simulink model "c00011M_harness"  (R2018a)
settings: Solver=FixedStepAuto  StartTime=0.0  StopTime=300  FixedStep=0.1  RelTol=1e-3
undefined symbols (not defined in the file): A1, hmax, PriorityTank, R1, R2, sigbuilder_block
(part 10 of 73)

== system c00011M_harness/M145 ==
  note: VALUES
      | ---------------------------------
      | ControlType = 1 | 2 | 3
      | FillTank = 0 | 1
      | EmptyTank = 0 | 1
      | ManualReference between 0 and 1
      | Tempreature between 0 and 100
      | EmergencyButton = 0 | 1
      | LiquidLevel between 0 and 1 (hmax)
  note: Inputs For Tank2
  note: NAMES
      | --------------------------------------------
      | CT1 = ControlType Tank 1
      | F1 = Fill Tank 1
      | E1 = Empty Tank 1
      | MR1 = Manual Reference Tank1
      | T1 = Temperature Tank 1
      | EB1 = Emergency Button Tank 1
      | LL1 = Liquid Level 1
  note: Inputs For Tank3
  note: Inputs For Tank1
  CT1 : Inport
  MR1 : Inport  Port=2
  T1 : Inport  Port=3
  EB1 : Inport  Port=4
  CT2 : Inport  Port=5
  MR2 : Inport  Port=6
  T2 : Inport  Port=7
  EB2 : Inport  Port=8
  CT3 : Inport  Port=9
  F3 : Inport  Port=10
  E3 : Inport  Port=11
  T3 : Inport  Port=12
  EB3 : Inport  Port=13
  Tank1 : Subsystem
  Tank2 : Subsystem
  Tank3 : Subsystem
  LL1 : Outport
  LL2 : Outport  Port=2
  LL3 : Outport  Port=3
  wires:
  EB1/1 -> Tank1/4(EB1)
  Tank2/1(LL2) -> LL2/1, Tank3/7(LL2), Tank1/5(LL2)
  Tank3/1(LL3) -> LL3/1, Tank2/6(LL3), Tank1/6(LL3)
  EB2/1 -> Tank2/4(EB2)
  CT2/1 -> Tank2/1(CT2)
  MR1/1 -> Tank1/2(MR1)
  T1/1 -> Tank1/3(T1)
  Tank1/1(LL1) -> LL1/1, Tank3/6(LL1), Tank2/5(LL1)
  E3/1 -> Tank3/3(E3)
  T2/1 -> Tank2/3(T2)
  CT3/1 -> Tank3/1(CT3)
  F3/1 -> Tank3/2(F3)
  EB3/1 -> Tank3/5(EB3)
  T3/1 -> Tank3/4(T3)
  CT1/1 -> Tank1/1(CT1)
  MR2/1 -> Tank2/2(MR2)

== system c00011M_harness/M146 ==
  note: VALUES
      | ---------------------------------
      | ControlType = 1 | 2 | 3
      | FillTank = 0 | 1
      | EmptyTank = 0 | 1
      | ManualReference between 0 and 1
      | Tempreature between 0 and 100
      | EmergencyButton = 0 | 1
      | LiquidLevel between 0 and 1 (hmax)
  note: Inputs For Tank2
  note: NAMES
      | --------------------------------------------
      | CT1 = ControlType Tank 1
      | F1 = Fill Tank 1
      | E1 = Empty Tank 1
      | MR1 = Manual Reference Tank1
      | T1 = Temperature Tank 1
      | EB1 = Emergency Button Tank 1
      | LL1 = Liquid Level 1
  note: Inputs For Tank3
  note: Inputs For Tank1
  CT1 : Inport
  MR1 : Inport  Port=2
  T1 : Inport  Port=3
  EB1 : Inport  Port=4
  CT2 : Inport  Port=5
  MR2 : Inport  Port=6
  T2 : Inport  Port=7
  EB2 : Inport  Port=8
  CT3 : Inport  Port=9
  F3 : Inport  Port=10
  E3 : Inport  Port=11
  T3 : Inport  Port=12
  EB3 : Inport  Port=13
  Tank1 : Subsystem
  Tank2 : Subsystem
  Tank3 : Subsystem
  LL1 : Outport
  LL2 : Outport  Port=2
  LL3 : Outport  Port=3
  wires:
  EB1/1 -> Tank1/4(EB1)
  Tank2/1(LL2) -> LL2/1, Tank3/7(LL2), Tank1/5(LL2)
  Tank3/1(LL3) -> LL3/1, Tank2/6(LL3), Tank1/6(LL3)
  EB2/1 -> Tank2/4(EB2)
  CT2/1 -> Tank2/1(CT2)
  MR1/1 -> Tank1/2(MR1)
  T1/1 -> Tank1/3(T1)
  Tank1/1(LL1) -> LL1/1, Tank3/6(LL1), Tank2/5(LL1)
  E3/1 -> Tank3/3(E3)
  T2/1 -> Tank2/3(T2)
  CT3/1 -> Tank3/1(CT3)
  F3/1 -> Tank3/2(F3)
  EB3/1 -> Tank3/5(EB3)
  T3/1 -> Tank3/4(T3)
  CT1/1 -> Tank1/1(CT1)
  MR2/1 -> Tank2/2(MR2)

== system c00011M_harness/M147 ==
  note: VALUES
      | ---------------------------------
      | ControlType = 1 | 2 | 3
      | FillTank = 0 | 1
      | EmptyTank = 0 | 1
      | ManualReference between 0 and 1
      | Tempreature between 0 and 100
      | EmergencyButton = 0 | 1
      | LiquidLevel between 0 and 1 (hmax)
  note: Inputs For Tank2
  note: NAMES
      | --------------------------------------------
      | CT1 = ControlType Tank 1
      | F1 = Fill Tank 1
      | E1 = Empty Tank 1
      | MR1 = Manual Reference Tank1
      | T1 = Temperature Tank 1
      | EB1 = Emergency Button Tank 1
      | LL1 = Liquid Level 1
  note: Inputs For Tank3
  note: Inputs For Tank1
  CT1 : Inport
  MR1 : Inport  Port=2
  T1 : Inport  Port=3
  EB1 : Inport  Port=4
  CT2 : Inport  Port=5
  MR2 : Inport  Port=6
  T2 : Inport  Port=7
  EB2 : Inport  Port=8
  CT3 : Inport  Port=9
  F3 : Inport  Port=10
  E3 : Inport  Port=11
  T3 : Inport  Port=12
  EB3 : Inport  Port=13
  Tank1 : Subsystem
  Tank2 : Subsystem
  Tank3 : Subsystem
  LL1 : Outport
  LL2 : Outport  Port=2
  LL3 : Outport  Port=3
  wires:
  EB1/1 -> Tank1/4(EB1)
  Tank2/1(LL2) -> LL2/1, Tank3/7(LL2), Tank1/5(LL2)
  Tank3/1(LL3) -> LL3/1, Tank2/6(LL3), Tank1/6(LL3)
  EB2/1 -> Tank2/4(EB2)
  CT2/1 -> Tank2/1(CT2)
  MR1/1 -> Tank1/2(MR1)
  T1/1 -> Tank1/3(T1)
  Tank1/1(LL1) -> LL1/1, Tank3/6(LL1), Tank2/5(LL1)
  E3/1 -> Tank3/3(E3)
  T2/1 -> Tank2/3(T2)
  CT3/1 -> Tank3/1(CT3)
  F3/1 -> Tank3/2(F3)
  EB3/1 -> Tank3/5(EB3)
  T3/1 -> Tank3/4(T3)
  CT1/1 -> Tank1/1(CT1)
  MR2/1 -> Tank2/2(MR2)

== system c00011M_harness/M148 ==
  note: VALUES
      | ---------------------------------
      | ControlType = 1 | 2 | 3
      | FillTank = 0 | 1
      | EmptyTank = 0 | 1
      | ManualReference between 0 and 1
      | Tempreature between 0 and 100
      | EmergencyButton = 0 | 1
      | LiquidLevel between 0 and 1 (hmax)
  note: Inputs For Tank2
  note: NAMES
      | --------------------------------------------
      | CT1 = ControlType Tank 1
      | F1 = Fill Tank 1
      | E1 = Empty Tank 1
      | MR1 = Manual Reference Tank1
      | T1 = Temperature Tank 1
      | EB1 = Emergency Button Tank 1
      | LL1 = Liquid Level 1
  note: Inputs For Tank3
  note: Inputs For Tank1
  CT1 : Inport
  MR1 : Inport  Port=2
  T1 : Inport  Port=3
  EB1 : Inport  Port=4
  CT2 : Inport  Port=5
  MR2 : Inport  Port=6
  T2 : Inport  Port=7
  EB2 : Inport  Port=8
  CT3 : Inport  Port=9
  F3 : Inport  Port=10
  E3 : Inport  Port=11
  T3 : Inport  Port=12
  EB3 : Inport  Port=13
  Tank1 : Subsystem
  Tank2 : Subsystem
  Tank3 : Subsystem
  LL1 : Outport
  LL2 : Outport  Port=2
  LL3 : Outport  Port=3
  wires:
  EB1/1 -> Tank1/4(EB1)
  Tank2/1(LL2) -> LL2/1, Tank3/7(LL2), Tank1/5(LL2)
  Tank3/1(LL3) -> LL3/1, Tank2/6(LL3), Tank1/6(LL3)
  EB2/1 -> Tank2/4(EB2)
  CT2/1 -> Tank2/1(CT2)
  MR1/1 -> Tank1/2(MR1)
  T1/1 -> Tank1/3(T1)
  Tank1/1(LL1) -> LL1/1, Tank3/6(LL1), Tank2/5(LL1)
  E3/1 -> Tank3/3(E3)
  T2/1 -> Tank2/3(T2)
  CT3/1 -> Tank3/1(CT3)
  F3/1 -> Tank3/2(F3)
  EB3/1 -> Tank3/5(EB3)
  T3/1 -> Tank3/4(T3)
  CT1/1 -> Tank1/1(CT1)
  MR2/1 -> Tank2/2(MR2)

== system c00011M_harness/M149 ==
  note: VALUES
      | ---------------------------------
      | ControlType = 1 | 2 | 3
      | FillTank = 0 | 1
      | EmptyTank = 0 | 1
      | ManualReference between 0 and 1
      | Tempreature between 0 and 100
      | EmergencyButton = 0 | 1
      | LiquidLevel between 0 and 1 (hmax)
  note: Inputs For Tank2
  note: NAMES
      | --------------------------------------------
      | CT1 = ControlType Tank 1
      | F1 = Fill Tank 1
      | E1 = Empty Tank 1
      | MR1 = Manual Reference Tank1
      | T1 = Temperature Tank 1
      | EB1 = Emergency Button Tank 1
      | LL1 = Liquid Level 1
  note: Inputs For Tank3
  note: Inputs For Tank1
  CT1 : Inport
  MR1 : Inport  Port=2
  T1 : Inport  Port=3
  EB1 : Inport  Port=4
  CT2 : Inport  Port=5
  MR2 : Inport  Port=6
  T2 : Inport  Port=7
  EB2 : Inport  Port=8
  CT3 : Inport  Port=9
  F3 : Inport  Port=10
  E3 : Inport  Port=11
  T3 : Inport  Port=12
  EB3 : Inport  Port=13
  Tank1 : Subsystem
  Tank2 : Subsystem
  Tank3 : Subsystem
  LL1 : Outport
  LL2 : Outport  Port=2
  LL3 : Outport  Port=3
  wires:
  EB1/1 -> Tank1/4(EB1)
  Tank2/1(LL2) -> LL2/1, Tank3/7(LL2), Tank1/5(LL2)
  Tank3/1(LL3) -> LL3/1, Tank2/6(LL3), Tank1/6(LL3)
  EB2/1 -> Tank2/4(EB2)
  CT2/1 -> Tank2/1(CT2)
  MR1/1 -> Tank1/2(MR1)
  T1/1 -> Tank1/3(T1)
  Tank1/1(LL1) -> LL1/1, Tank3/6(LL1), Tank2/5(LL1)
  E3/1 -> Tank3/3(E3)
  T2/1 -> Tank2/3(T2)
  CT3/1 -> Tank3/1(CT3)
  F3/1 -> Tank3/2(F3)
  EB3/1 -> Tank3/5(EB3)
  T3/1 -> Tank3/4(T3)
  CT1/1 -> Tank1/1(CT1)
  MR2/1 -> Tank2/2(MR2)

== system c00011M_harness/M150 ==
  note: VALUES
      | ---------------------------------
      | ControlType = 1 | 2 | 3
      | FillTank = 0 | 1
      | EmptyTank = 0 | 1
      | ManualReference between 0 and 1
      | Tempreature between 0 and 100
      | EmergencyButton = 0 | 1
      | LiquidLevel between 0 and 1 (hmax)
  note: Inputs For Tank2
  note: NAMES
      | --------------------------------------------
      | CT1 = ControlType Tank 1
      | F1 = Fill Tank 1
      | E1 = Empty Tank 1
      | MR1 = Manual Reference Tank1
      | T1 = Temperature Tank 1
      | EB1 = Emergency Button Tank 1
      | LL1 = Liquid Level 1
  note: Inputs For Tank3
  note: Inputs For Tank1
  CT1 : Inport
  MR1 : Inport  Port=2
  T1 : Inport  Port=3
  EB1 : Inport  Port=4
  CT2 : Inport  Port=5
  MR2 : Inport  Port=6
  T2 : Inport  Port=7
  EB2 : Inport  Port=8
  CT3 : Inport  Port=9
  F3 : Inport  Port=10
  E3 : Inport  Port=11
  T3 : Inport  Port=12
  EB3 : Inport  Port=13
  Tank1 : Subsystem
  Tank2 : Subsystem
  Tank3 : Subsystem
  LL1 : Outport
  LL2 : Outport  Port=2
  LL3 : Outport  Port=3
  wires:
  EB1/1 -> Tank1/4(EB1)
  Tank2/1(LL2) -> LL2/1, Tank3/7(LL2), Tank1/5(LL2)
  Tank3/1(LL3) -> LL3/1, Tank2/6(LL3), Tank1/6(LL3)
  EB2/1 -> Tank2/4(EB2)
  CT2/1 -> Tank2/1(CT2)
  MR1/1 -> Tank1/2(MR1)
  T1/1 -> Tank1/3(T1)
  Tank1/1(LL1) -> LL1/1, Tank3/6(LL1), Tank2/5(LL1)
  E3/1 -> Tank3/3(E3)
  T2/1 -> Tank2/3(T2)
  CT3/1 -> Tank3/1(CT3)
  F3/1 -> Tank3/2(F3)
  EB3/1 -> Tank3/5(EB3)
  T3/1 -> Tank3/4(T3)
  CT1/1 -> Tank1/1(CT1)
  MR2/1 -> Tank2/2(MR2)

== system c00011M_harness/M151 ==
  note: VALUES
      | ---------------------------------
      | ControlType = 1 | 2 | 3
      | FillTank = 0 | 1
      | EmptyTank = 0 | 1
      | ManualReference between 0 and 1
      | Tempreature between 0 and 100
      | EmergencyButton = 0 | 1
      | LiquidLevel between 0 and 1 (hmax)
  note: Inputs For Tank2
  note: NAMES
      | --------------------------------------------
      | CT1 = ControlType Tank 1
      | F1 = Fill Tank 1
      | E1 = Empty Tank 1
      | MR1 = Manual Reference Tank1
      | T1 = Temperature Tank 1
      | EB1 = Emergency Button Tank 1
      | LL1 = Liquid Level 1
  note: Inputs For Tank3
  note: Inputs For Tank1
  CT1 : Inport
  MR1 : Inport  Port=2
  T1 : Inport  Port=3
  EB1 : Inport  Port=4
  CT2 : Inport  Port=5
  MR2 : Inport  Port=6
  T2 : Inport  Port=7
  EB2 : Inport  Port=8
  CT3 : Inport  Port=9
  F3 : Inport  Port=10
  E3 : Inport  Port=11
  T3 : Inport  Port=12
  EB3 : Inport  Port=13
  Tank1 : Subsystem
  Tank2 : Subsystem
  Tank3 : Subsystem
  LL1 : Outport
  LL2 : Outport  Port=2
  LL3 : Outport  Port=3
  wires:
  EB1/1 -> Tank1/4(EB1)
  Tank2/1(LL2) -> LL2/1, Tank3/7(LL2), Tank1/5(LL2)
  Tank3/1(LL3) -> LL3/1, Tank2/6(LL3), Tank1/6(LL3)
  EB2/1 -> Tank2/4(EB2)
  CT2/1 -> Tank2/1(CT2)
  MR1/1 -> Tank1/2(MR1)
  T1/1 -> Tank1/3(T1)
  Tank1/1(LL1) -> LL1/1, Tank3/6(LL1), Tank2/5(LL1)
  E3/1 -> Tank3/3(E3)
  T2/1 -> Tank2/3(T2)
  CT3/1 -> Tank3/1(CT3)
  F3/1 -> Tank3/2(F3)
  EB3/1 -> Tank3/5(EB3)
  T3/1 -> Tank3/4(T3)
  CT1/1 -> Tank1/1(CT1)
  MR2/1 -> Tank2/2(MR2)

== system c00011M_harness/M152 ==
  note: VALUES
      | ---------------------------------
      | ControlType = 1 | 2 | 3
      | FillTank = 0 | 1
      | EmptyTank = 0 | 1
      | ManualReference between 0 and 1
      | Tempreature between 0 and 100
      | EmergencyButton = 0 | 1
      | LiquidLevel between 0 and 1 (hmax)
  note: Inputs For Tank2
  note: NAMES
      | --------------------------------------------
      | CT1 = ControlType Tank 1
      | F1 = Fill Tank 1
      | E1 = Empty Tank 1
      | MR1 = Manual Reference Tank1
      | T1 = Temperature Tank 1
      | EB1 = Emergency Button Tank 1
      | LL1 = Liquid Level 1
  note: Inputs For Tank3
  note: Inputs For Tank1
  CT1 : Inport
  MR1 : Inport  Port=2
  T1 : Inport  Port=3
  EB1 : Inport  Port=4
  CT2 : Inport  Port=5
  MR2 : Inport  Port=6
  T2 : Inport  Port=7
  EB2 : Inport  Port=8
  CT3 : Inport  Port=9
  F3 : Inport  Port=10
  E3 : Inport  Port=11
  T3 : Inport  Port=12
  EB3 : Inport  Port=13
  Tank1 : Subsystem
  Tank2 : Subsystem
  Tank3 : Subsystem
  LL1 : Outport
  LL2 : Outport  Port=2
  LL3 : Outport  Port=3
  wires:
  EB1/1 -> Tank1/4(EB1)
  Tank2/1(LL2) -> LL2/1, Tank3/7(LL2), Tank1/5(LL2)
  Tank3/1(LL3) -> LL3/1, Tank2/6(LL3), Tank1/6(LL3)
  EB2/1 -> Tank2/4(EB2)
  CT2/1 -> Tank2/1(CT2)
  MR1/1 -> Tank1/2(MR1)
  T1/1 -> Tank1/3(T1)
  Tank1/1(LL1) -> LL1/1, Tank3/6(LL1), Tank2/5(LL1)
  E3/1 -> Tank3/3(E3)
  T2/1 -> Tank2/3(T2)
  CT3/1 -> Tank3/1(CT3)
  F3/1 -> Tank3/2(F3)
  EB3/1 -> Tank3/5(EB3)
  T3/1 -> Tank3/4(T3)
  CT1/1 -> Tank1/1(CT1)
  MR2/1 -> Tank2/2(MR2)

== system c00011M_harness/M153 ==
  note: VALUES
      | ---------------------------------
      | ControlType = 1 | 2 | 3
      | FillTank = 0 | 1
      | EmptyTank = 0 | 1
      | ManualReference between 0 and 1
      | Tempreature between 0 and 100
      | EmergencyButton = 0 | 1
      | LiquidLevel between 0 and 1 (hmax)
  note: Inputs For Tank2
  note: NAMES
      | --------------------------------------------
      | CT1 = ControlType Tank 1
      | F1 = Fill Tank 1
      | E1 = Empty Tank 1
      | MR1 = Manual Reference Tank1
      | T1 = Temperature Tank 1
      | EB1 = Emergency Button Tank 1
      | LL1 = Liquid Level 1
  note: Inputs For Tank3
  note: Inputs For Tank1
  CT1 : Inport
  MR1 : Inport  Port=2
  T1 : Inport  Port=3
  EB1 : Inport  Port=4
  CT2 : Inport  Port=5
  MR2 : Inport  Port=6
  T2 : Inport  Port=7
  EB2 : Inport  Port=8
  CT3 : Inport  Port=9
  F3 : Inport  Port=10
  E3 : Inport  Port=11
  T3 : Inport  Port=12
  EB3 : Inport  Port=13
  Tank1 : Subsystem
  Tank2 : Subsystem
  Tank3 : Subsystem
  LL1 : Outport
  LL2 : Outport  Port=2
  LL3 : Outport  Port=3
  wires:
  EB1/1 -> Tank1/4(EB1)
  Tank2/1(LL2) -> LL2/1, Tank3/7(LL2), Tank1/5(LL2)
  Tank3/1(LL3) -> LL3/1, Tank2/6(LL3), Tank1/6(LL3)
  EB2/1 -> Tank2/4(EB2)
  CT2/1 -> Tank2/1(CT2)
  MR1/1 -> Tank1/2(MR1)
  T1/1 -> Tank1/3(T1)
  Tank1/1(LL1) -> LL1/1, Tank3/6(LL1), Tank2/5(LL1)
  E3/1 -> Tank3/3(E3)
  T2/1 -> Tank2/3(T2)
  CT3/1 -> Tank3/1(CT3)
  F3/1 -> Tank3/2(F3)
  EB3/1 -> Tank3/5(EB3)
  T3/1 -> Tank3/4(T3)
  CT1/1 -> Tank1/1(CT1)
  MR2/1 -> Tank2/2(MR2)

== system c00011M_harness/M154 ==
  note: VALUES
      | ---------------------------------
      | ControlType = 1 | 2 | 3
      | FillTank = 0 | 1
      | EmptyTank = 0 | 1
      | ManualReference between 0 and 1
      | Tempreature between 0 and 100
      | EmergencyButton = 0 | 1
      | LiquidLevel between 0 and 1 (hmax)
  note: Inputs For Tank2
  note: NAMES
      | --------------------------------------------
      | CT1 = ControlType Tank 1
      | F1 = Fill Tank 1
      | E1 = Empty Tank 1
      | MR1 = Manual Reference Tank1
      | T1 = Temperature Tank 1
      | EB1 = Emergency Button Tank 1
      | LL1 = Liquid Level 1
  note: Inputs For Tank3
  note: Inputs For Tank1
  CT1 : Inport
  MR1 : Inport  Port=2
  T1 : Inport  Port=3
  EB1 : Inport  Port=4
  CT2 : Inport  Port=5
  MR2 : Inport  Port=6
  T2 : Inport  Port=7
  EB2 : Inport  Port=8
  CT3 : Inport  Port=9
  F3 : Inport  Port=10
  E3 : Inport  Port=11
  T3 : Inport  Port=12
  EB3 : Inport  Port=13
  Tank1 : Subsystem
  Tank2 : Subsystem
  Tank3 : Subsystem
  LL1 : Outport
  LL2 : Outport  Port=2
  LL3 : Outport  Port=3
  wires:
  EB1/1 -> Tank1/4(EB1)
  Tank2/1(LL2) -> LL2/1, Tank3/7(LL2), Tank1/5(LL2)
  Tank3/1(LL3) -> LL3/1, Tank2/6(LL3), Tank1/6(LL3)
  EB2/1 -> Tank2/4(EB2)
  CT2/1 -> Tank2/1(CT2)
  MR1/1 -> Tank1/2(MR1)
  T1/1 -> Tank1/3(T1)
  Tank1/1(LL1) -> LL1/1, Tank3/6(LL1), Tank2/5(LL1)
  E3/1 -> Tank3/3(E3)
  T2/1 -> Tank2/3(T2)
  CT3/1 -> Tank3/1(CT3)
  F3/1 -> Tank3/2(F3)
  EB3/1 -> Tank3/5(EB3)
  T3/1 -> Tank3/4(T3)
  CT1/1 -> Tank1/1(CT1)
  MR2/1 -> Tank2/2(MR2)

== system c00011M_harness/M155 ==
  note: VALUES
      | ---------------------------------
      | ControlType = 1 | 2 | 3
      | FillTank = 0 | 1
      | EmptyTank = 0 | 1
      | ManualReference between 0 and 1
      | Tempreature between 0 and 100
      | EmergencyButton = 0 | 1
      | LiquidLevel between 0 and 1 (hmax)
  note: Inputs For Tank2
  note: NAMES
      | --------------------------------------------
      | CT1 = ControlType Tank 1
      | F1 = Fill Tank 1
      | E1 = Empty Tank 1
      | MR1 = Manual Reference Tank1
      | T1 = Temperature Tank 1
      | EB1 = Emergency Button Tank 1
      | LL1 = Liquid Level 1
  note: Inputs For Tank3
  note: Inputs For Tank1
  CT1 : Inport
  MR1 : Inport  Port=2
  T1 : Inport  Port=3
  EB1 : Inport  Port=4
  CT2 : Inport  Port=5
  MR2 : Inport  Port=6
  T2 : Inport  Port=7
  EB2 : Inport  Port=8
  CT3 : Inport  Port=9
  F3 : Inport  Port=10
  E3 : Inport  Port=11
  T3 : Inport  Port=12
  EB3 : Inport  Port=13
  Tank1 : Subsystem
  Tank2 : Subsystem
  Tank3 : Subsystem
  LL1 : Outport
  LL2 : Outport  Port=2
  LL3 : Outport  Port=3
  wires:
  EB1/1 -> Tank1/4(EB1)
  Tank2/1(LL2) -> LL2/1, Tank3/7(LL2), Tank1/5(LL2)
  Tank3/1(LL3) -> LL3/1, Tank2/6(LL3), Tank1/6(LL3)
  EB2/1 -> Tank2/4(EB2)
  CT2/1 -> Tank2/1(CT2)
  MR1/1 -> Tank1/2(MR1)
  T1/1 -> Tank1/3(T1)
  Tank1/1(LL1) -> LL1/1, Tank3/6(LL1), Tank2/5(LL1)
  E3/1 -> Tank3/3(E3)
  T2/1 -> Tank2/3(T2)
  CT3/1 -> Tank3/1(CT3)
  F3/1 -> Tank3/2(F3)
  EB3/1 -> Tank3/5(EB3)
  T3/1 -> Tank3/4(T3)
  CT1/1 -> Tank1/1(CT1)
  MR2/1 -> Tank2/2(MR2)

== system c00011M_harness/M156 ==
  note: VALUES
      | ---------------------------------
      | ControlType = 1 | 2 | 3
      | FillTank = 0 | 1
      | EmptyTank = 0 | 1
      | ManualReference between 0 and 1
      | Tempreature between 0 and 100
      | EmergencyButton = 0 | 1
      | LiquidLevel between 0 and 1 (hmax)
  note: Inputs For Tank2
  note: NAMES
      | --------------------------------------------
      | CT1 = ControlType Tank 1
      | F1 = Fill Tank 1
      | E1 = Empty Tank 1
      | MR1 = Manual Reference Tank1
      | T1 = Temperature Tank 1
      | EB1 = Emergency Button Tank 1
      | LL1 = Liquid Level 1
  note: Inputs For Tank3
  note: Inputs For Tank1
  CT1 : Inport
  MR1 : Inport  Port=2
  T1 : Inport  Port=3
  EB1 : Inport  Port=4
  CT2 : Inport  Port=5
  MR2 : Inport  Port=6
  T2 : Inport  Port=7
  EB2 : Inport  Port=8
  CT3 : Inport  Port=9
  F3 : Inport  Port=10
  E3 : Inport  Port=11
  T3 : Inport  Port=12
  EB3 : Inport  Port=13
  Tank1 : Subsystem
  Tank2 : Subsystem
  Tank3 : Subsystem
  LL1 : Outport
  LL2 : Outport  Port=2
  LL3 : Outport  Port=3
  wires:
  EB1/1 -> Tank1/4(EB1)
  Tank2/1(LL2) -> LL2/1, Tank3/7(LL2), Tank1/5(LL2)
  Tank3/1(LL3) -> LL3/1, Tank2/6(LL3), Tank1/6(LL3)
  EB2/1 -> Tank2/4(EB2)
  CT2/1 -> Tank2/1(CT2)
  MR1/1 -> Tank1/2(MR1)
  T1/1 -> Tank1/3(T1)
  Tank1/1(LL1) -> LL1/1, Tank3/6(LL1), Tank2/5(LL1)
  E3/1 -> Tank3/3(E3)
  T2/1 -> Tank2/3(T2)
  CT3/1 -> Tank3/1(CT3)
  F3/1 -> Tank3/2(F3)
  EB3/1 -> Tank3/5(EB3)
  T3/1 -> Tank3/4(T3)
  CT1/1 -> Tank1/1(CT1)
  MR2/1 -> Tank2/2(MR2)

== system c00011M_harness/M157 ==
  note: VALUES
      | ---------------------------------
      | ControlType = 1 | 2 | 3
      | FillTank = 0 | 1
      | EmptyTank = 0 | 1
      | ManualReference between 0 and 1
      | Tempreature between 0 and 100
      | EmergencyButton = 0 | 1
      | LiquidLevel between 0 and 1 (hmax)
  note: Inputs For Tank2
  note: NAMES
      | --------------------------------------------
      | CT1 = ControlType Tank 1
      | F1 = Fill Tank 1
      | E1 = Empty Tank 1
      | MR1 = Manual Reference Tank1
      | T1 = Temperature Tank 1
      | EB1 = Emergency Button Tank 1
      | LL1 = Liquid Level 1
  note: Inputs For Tank3
  note: Inputs For Tank1
  CT1 : Inport
  MR1 : Inport  Port=2
  T1 : Inport  Port=3
  EB1 : Inport  Port=4
  CT2 : Inport  Port=5
  MR2 : Inport  Port=6
  T2 : Inport  Port=7
  EB2 : Inport  Port=8
  CT3 : Inport  Port=9
  F3 : Inport  Port=10
  E3 : Inport  Port=11
  T3 : Inport  Port=12
  EB3 : Inport  Port=13
  Tank1 : Subsystem
  Tank2 : Subsystem
  Tank3 : Subsystem
  LL1 : Outport
  LL2 : Outport  Port=2
  LL3 : Outport  Port=3
  wires:
  EB1/1 -> Tank1/4(EB1)
  Tank2/1(LL2) -> LL2/1, Tank3/7(LL2), Tank1/5(LL2)
  Tank3/1(LL3) -> LL3/1, Tank2/6(LL3), Tank1/6(LL3)
  EB2/1 -> Tank2/4(EB2)
  CT2/1 -> Tank2/1(CT2)
  MR1/1 -> Tank1/2(MR1)
  T1/1 -> Tank1/3(T1)
  Tank1/1(LL1) -> LL1/1, Tank3/6(LL1), Tank2/5(LL1)
  E3/1 -> Tank3/3(E3)
  T2/1 -> Tank2/3(T2)
  CT3/1 -> Tank3/1(CT3)
  F3/1 -> Tank3/2(F3)
  EB3/1 -> Tank3/5(EB3)
  T3/1 -> Tank3/4(T3)
  CT1/1 -> Tank1/1(CT1)
  MR2/1 -> Tank2/2(MR2)

== system c00011M_harness/M158 ==
  note: VALUES
      | ---------------------------------
      | ControlType = 1 | 2 | 3
      | FillTank = 0 | 1
      | EmptyTank = 0 | 1
      | ManualReference between 0 and 1
      | Tempreature between 0 and 100
      | EmergencyButton = 0 | 1
      | LiquidLevel between 0 and 1 (hmax)
  note: Inputs For Tank2
  note: NAMES
      | --------------------------------------------
      | CT1 = ControlType Tank 1
      | F1 = Fill Tank 1
      | E1 = Empty Tank 1
      | MR1 = Manual Reference Tank1
      | T1 = Temperature Tank 1
      | EB1 = Emergency Button Tank 1
      | LL1 = Liquid Level 1
  note: Inputs For Tank3
  note: Inputs For Tank1
  CT1 : Inport
  MR1 : Inport  Port=2
  T1 : Inport  Port=3
  EB1 : Inport  Port=4
  CT2 : Inport  Port=5
  MR2 : Inport  Port=6
  T2 : Inport  Port=7
  EB2 : Inport  Port=8
  CT3 : Inport  Port=9
  F3 : Inport  Port=10
  E3 : Inport  Port=11
  T3 : Inport  Port=12
  EB3 : Inport  Port=13
  Tank1 : Subsystem
  Tank2 : Subsystem
  Tank3 : Subsystem
  LL1 : Outport
  LL2 : Outport  Port=2
  LL3 : Outport  Port=3
  wires:
  EB1/1 -> Tank1/4(EB1)
  Tank2/1(LL2) -> LL2/1, Tank3/7(LL2), Tank1/5(LL2)
  Tank3/1(LL3) -> LL3/1, Tank2/6(LL3), Tank1/6(LL3)
  EB2/1 -> Tank2/4(EB2)
  CT2/1 -> Tank2/1(CT2)
  MR1/1 -> Tank1/2(MR1)
  T1/1 -> Tank1/3(T1)
  Tank1/1(LL1) -> LL1/1, Tank3/6(LL1), Tank2/5(LL1)
  E3/1 -> Tank3/3(E3)
  T2/1 -> Tank2/3(T2)
  CT3/1 -> Tank3/1(CT3)
  F3/1 -> Tank3/2(F3)
  EB3/1 -> Tank3/5(EB3)
  T3/1 -> Tank3/4(T3)
  CT1/1 -> Tank1/1(CT1)
  MR2/1 -> Tank2/2(MR2)

== system c00011M_harness/M159 ==
  note: VALUES
      | ---------------------------------
      | ControlType = 1 | 2 | 3
      | FillTank = 0 | 1
      | EmptyTank = 0 | 1
      | ManualReference between 0 and 1
      | Tempreature between 0 and 100
      | EmergencyButton = 0 | 1
      | LiquidLevel between 0 and 1 (hmax)
  note: Inputs For Tank2
  note: NAMES
      | --------------------------------------------
      | CT1 = ControlType Tank 1
      | F1 = Fill Tank 1
      | E1 = Empty Tank 1
      | MR1 = Manual Reference Tank1
      | T1 = Temperature Tank 1
      | EB1 = Emergency Button Tank 1
      | LL1 = Liquid Level 1
  note: Inputs For Tank3
  note: Inputs For Tank1
  CT1 : Inport
  MR1 : Inport  Port=2
  T1 : Inport  Port=3
  EB1 : Inport  Port=4
  CT2 : Inport  Port=5
  MR2 : Inport  Port=6
  T2 : Inport  Port=7
  EB2 : Inport  Port=8
  CT3 : Inport  Port=9
  F3 : Inport  Port=10
  E3 : Inport  Port=11
  T3 : Inport  Port=12
  EB3 : Inport  Port=13
  Tank1 : Subsystem
  Tank2 : Subsystem
  Tank3 : Subsystem
  LL1 : Outport
  LL2 : Outport  Port=2
  LL3 : Outport  Port=3
  wires:
  EB1/1 -> Tank1/4(EB1)
  Tank2/1(LL2) -> LL2/1, Tank3/7(LL2), Tank1/5(LL2)
  Tank3/1(LL3) -> LL3/1, Tank2/6(LL3), Tank1/6(LL3)
  EB2/1 -> Tank2/4(EB2)
  CT2/1 -> Tank2/1(CT2)
  MR1/1 -> Tank1/2(MR1)
  T1/1 -> Tank1/3(T1)
  Tank1/1(LL1) -> LL1/1, Tank3/6(LL1), Tank2/5(LL1)
  E3/1 -> Tank3/3(E3)
  T2/1 -> Tank2/3(T2)
  CT3/1 -> Tank3/1(CT3)
  F3/1 -> Tank3/2(F3)
  EB3/1 -> Tank3/5(EB3)
  T3/1 -> Tank3/4(T3)
  CT1/1 -> Tank1/1(CT1)
  MR2/1 -> Tank2/2(MR2)

== system c00011M_harness/M160 ==
  note: VALUES
      | ---------------------------------
      | ControlType = 1 | 2 | 3
      | FillTank = 0 | 1
      | EmptyTank = 0 | 1
      | ManualReference between 0 and 1
      | Tempreature between 0 and 100
      | EmergencyButton = 0 | 1
      | LiquidLevel between 0 and 1 (hmax)
  note: Inputs For Tank2
  note: NAMES
      | --------------------------------------------
      | CT1 = ControlType Tank 1
      | F1 = Fill Tank 1
      | E1 = Empty Tank 1
      | MR1 = Manual Reference Tank1
      | T1 = Temperature Tank 1
      | EB1 = Emergency Button Tank 1
      | LL1 = Liquid Level 1
  note: Inputs For Tank3
  note: Inputs For Tank1
  CT1 : Inport
  MR1 : Inport  Port=2
  T1 : Inport  Port=3
  EB1 : Inport  Port=4
  CT2 : Inport  Port=5
  MR2 : Inport  Port=6
  T2 : Inport  Port=7
  EB2 : Inport  Port=8
  CT3 : Inport  Port=9
  F3 : Inport  Port=10
  E3 : Inport  Port=11
  T3 : Inport  Port=12
  EB3 : Inport  Port=13
  Tank1 : Subsystem
  Tank2 : Subsystem
  Tank3 : Subsystem
  LL1 : Outport
  LL2 : Outport  Port=2
  LL3 : Outport  Port=3
  wires:
  EB1/1 -> Tank1/4(EB1)
  Tank2/1(LL2) -> LL2/1, Tank3/7(LL2), Tank1/5(LL2)
  Tank3/1(LL3) -> LL3/1, Tank2/6(LL3), Tank1/6(LL3)
  EB2/1 -> Tank2/4(EB2)
  CT2/1 -> Tank2/1(CT2)
  MR1/1 -> Tank1/2(MR1)
  T1/1 -> Tank1/3(T1)
  Tank1/1(LL1) -> LL1/1, Tank3/6(LL1), Tank2/5(LL1)
  E3/1 -> Tank3/3(E3)
  T2/1 -> Tank2/3(T2)
  CT3/1 -> Tank3/1(CT3)
  F3/1 -> Tank3/2(F3)
  EB3/1 -> Tank3/5(EB3)
  T3/1 -> Tank3/4(T3)
  CT1/1 -> Tank1/1(CT1)
  MR2/1 -> Tank2/2(MR2)

== system c00011M_harness/M161 ==
  note: VALUES
      | ---------------------------------
      | ControlType = 1 | 2 | 3
      | FillTank = 0 | 1
      | EmptyTank = 0 | 1
      | ManualReference between 0 and 1
      | Tempreature between 0 and 100
      | EmergencyButton = 0 | 1
      | LiquidLevel between 0 and 1 (hmax)
  note: Inputs For Tank2
  note: NAMES
      | --------------------------------------------
      | CT1 = ControlType Tank 1
      | F1 = Fill Tank 1
      | E1 = Empty Tank 1
      | MR1 = Manual Reference Tank1
      | T1 = Temperature Tank 1
      | EB1 = Emergency Button Tank 1
      | LL1 = Liquid Level 1
  note: Inputs For Tank3
  note: Inputs For Tank1
  CT1 : Inport
  MR1 : Inport  Port=2
  T1 : Inport  Port=3
  EB1 : Inport  Port=4
  CT2 : Inport  Port=5
  MR2 : Inport  Port=6
  T2 : Inport  Port=7
  EB2 : Inport  Port=8
  CT3 : Inport  Port=9
  F3 : Inport  Port=10
  E3 : Inport  Port=11
  T3 : Inport  Port=12
  EB3 : Inport  Port=13
  Tank1 : Subsystem
  Tank2 : Subsystem
  Tank3 : Subsystem
  LL1 : Outport
  LL2 : Outport  Port=2
  LL3 : Outport  Port=3
  wires:
  EB1/1 -> Tank1/4(EB1)
  Tank2/1(LL2) -> LL2/1, Tank3/7(LL2), Tank1/5(LL2)
  Tank3/1(LL3) -> LL3/1, Tank2/6(LL3), Tank1/6(LL3)
  EB2/1 -> Tank2/4(EB2)
  CT2/1 -> Tank2/1(CT2)
  MR1/1 -> Tank1/2(MR1)
  T1/1 -> Tank1/3(T1)
  Tank1/1(LL1) -> LL1/1, Tank3/6(LL1), Tank2/5(LL1)
  E3/1 -> Tank3/3(E3)
  T2/1 -> Tank2/3(T2)
  CT3/1 -> Tank3/1(CT3)
  F3/1 -> Tank3/2(F3)
  EB3/1 -> Tank3/5(EB3)
  T3/1 -> Tank3/4(T3)
  CT1/1 -> Tank1/1(CT1)
  MR2/1 -> Tank2/2(MR2)

== system c00011M_harness/M162 ==
  note: VALUES
      | ---------------------------------
      | ControlType = 1 | 2 | 3
      | FillTank = 0 | 1
      | EmptyTank = 0 | 1
      | ManualReference between 0 and 1
      | Tempreature between 0 and 100
      | EmergencyButton = 0 | 1
      | LiquidLevel between 0 and 1 (hmax)
  note: Inputs For Tank2
  note: NAMES
      | --------------------------------------------
      | CT1 = ControlType Tank 1
      | F1 = Fill Tank 1
      | E1 = Empty Tank 1
      | MR1 = Manual Reference Tank1
      | T1 = Temperature Tank 1
      | EB1 = Emergency Button Tank 1
      | LL1 = Liquid Level 1
  note: Inputs For Tank3
  note: Inputs For Tank1
  CT1 : Inport
  MR1 : Inport  Port=2
  T1 : Inport  Port=3
  EB1 : Inport  Port=4
  CT2 : Inport  Port=5
  MR2 : Inport  Port=6
  T2 : Inport  Port=7
  EB2 : Inport  Port=8
  CT3 : Inport  Port=9
  F3 : Inport  Port=10
  E3 : Inport  Port=11
  T3 : Inport  Port=12
  EB3 : Inport  Port=13
  Tank1 : Subsystem
  Tank2 : Subsystem
  Tank3 : Subsystem
  LL1 : Outport
  LL2 : Outport  Port=2
  LL3 : Outport  Port=3
  wires:
  EB1/1 -> Tank1/4(EB1)
  Tank2/1(LL2) -> LL2/1, Tank3/7(LL2), Tank1/5(LL2)
  Tank3/1(LL3) -> LL3/1, Tank2/6(LL3), Tank1/6(LL3)
  EB2/1 -> Tank2/4(EB2)
  CT2/1 -> Tank2/1(CT2)
  MR1/1 -> Tank1/2(MR1)
  T1/1 -> Tank1/3(T1)
  Tank1/1(LL1) -> LL1/1, Tank3/6(LL1), Tank2/5(LL1)
  E3/1 -> Tank3/3(E3)
  T2/1 -> Tank2/3(T2)
  CT3/1 -> Tank3/1(CT3)
  F3/1 -> Tank3/2(F3)
  EB3/1 -> Tank3/5(EB3)
  T3/1 -> Tank3/4(T3)
  CT1/1 -> Tank1/1(CT1)
  MR2/1 -> Tank2/2(MR2)

== system c00011M_harness/M163 ==
  note: VALUES
      | ---------------------------------
      | ControlType = 1 | 2 | 3
      | FillTank = 0 | 1
      | EmptyTank = 0 | 1
      | ManualReference between 0 and 1
      | Tempreature between 0 and 100
      | EmergencyButton = 0 | 1
      | LiquidLevel between 0 and 1 (hmax)
  note: Inputs For Tank2
  note: NAMES
      | --------------------------------------------
      | CT1 = ControlType Tank 1
      | F1 = Fill Tank 1
      | E1 = Empty Tank 1
      | MR1 = Manual Reference Tank1
      | T1 = Temperature Tank 1
      | EB1 = Emergency Button Tank 1
      | LL1 = Liquid Level 1
  note: Inputs For Tank3
  note: Inputs For Tank1
  CT1 : Inport
  MR1 : Inport  Port=2
  T1 : Inport  Port=3
  EB1 : Inport  Port=4
  CT2 : Inport  Port=5
  MR2 : Inport  Port=6
  T2 : Inport  Port=7
  EB2 : Inport  Port=8
  CT3 : Inport  Port=9
  F3 : Inport  Port=10
  E3 : Inport  Port=11
  T3 : Inport  Port=12
  EB3 : Inport  Port=13
  Tank1 : Subsystem
  Tank2 : Subsystem
  Tank3 : Subsystem
  LL1 : Outport
  LL2 : Outport  Port=2
  LL3 : Outport  Port=3
  wires:
  EB1/1 -> Tank1/4(EB1)
  Tank2/1(LL2) -> LL2/1, Tank3/7(LL2), Tank1/5(LL2)
  Tank3/1(LL3) -> LL3/1, Tank2/6(LL3), Tank1/6(LL3)
  EB2/1 -> Tank2/4(EB2)
  CT2/1 -> Tank2/1(CT2)
  MR1/1 -> Tank1/2(MR1)
  T1/1 -> Tank1/3(T1)
  Tank1/1(LL1) -> LL1/1, Tank3/6(LL1), Tank2/5(LL1)
  E3/1 -> Tank3/3(E3)
  T2/1 -> Tank2/3(T2)
  CT3/1 -> Tank3/1(CT3)
  F3/1 -> Tank3/2(F3)
  EB3/1 -> Tank3/5(EB3)
  T3/1 -> Tank3/4(T3)
  CT1/1 -> Tank1/1(CT1)
  MR2/1 -> Tank2/2(MR2)

== system c00011M_harness/M164 ==
  note: VALUES
      | ---------------------------------
      | ControlType = 1 | 2 | 3
      | FillTank = 0 | 1
      | EmptyTank = 0 | 1
      | ManualReference between 0 and 1
      | Tempreature between 0 and 100
      | EmergencyButton = 0 | 1
      | LiquidLevel between 0 and 1 (hmax)
  note: Inputs For Tank2
  note: NAMES
      | --------------------------------------------
      | CT1 = ControlType Tank 1
      | F1 = Fill Tank 1
      | E1 = Empty Tank 1
      | MR1 = Manual Reference Tank1
      | T1 = Temperature Tank 1
      | EB1 = Emergency Button Tank 1
      | LL1 = Liquid Level 1
  note: Inputs For Tank3
  note: Inputs For Tank1
  CT1 : Inport
  MR1 : Inport  Port=2
  T1 : Inport  Port=3
  EB1 : Inport  Port=4
  CT2 : Inport  Port=5
  MR2 : Inport  Port=6
  T2 : Inport  Port=7
  EB2 : Inport  Port=8
  CT3 : Inport  Port=9
  F3 : Inport  Port=10
  E3 : Inport  Port=11
  T3 : Inport  Port=12
  EB3 : Inport  Port=13
  Tank1 : Subsystem
  Tank2 : Subsystem
  Tank3 : Subsystem
  LL1 : Outport
  LL2 : Outport  Port=2
  LL3 : Outport  Port=3
  wires:
  EB1/1 -> Tank1/4(EB1)
  Tank2/1(LL2) -> LL2/1, Tank3/7(LL2), Tank1/5(LL2)
  Tank3/1(LL3) -> LL3/1, Tank2/6(LL3), Tank1/6(LL3)
  EB2/1 -> Tank2/4(EB2)
  CT2/1 -> Tank2/1(CT2)
  MR1/1 -> Tank1/2(MR1)
  T1/1 -> Tank1/3(T1)
  Tank1/1(LL1) -> LL1/1, Tank3/6(LL1), Tank2/5(LL1)
  E3/1 -> Tank3/3(E3)
  T2/1 -> Tank2/3(T2)
  CT3/1 -> Tank3/1(CT3)
  F3/1 -> Tank3/2(F3)
  EB3/1 -> Tank3/5(EB3)
  T3/1 -> Tank3/4(T3)
  CT1/1 -> Tank1/1(CT1)
  MR2/1 -> Tank2/2(MR2)

== system c00011M_harness/M165 ==
  note: VALUES
      | ---------------------------------
      | ControlType = 1 | 2 | 3
      | FillTank = 0 | 1
      | EmptyTank = 0 | 1
      | ManualReference between 0 and 1
      | Tempreature between 0 and 100
      | EmergencyButton = 0 | 1
      | LiquidLevel between 0 and 1 (hmax)
  note: Inputs For Tank2
  note: NAMES
      | --------------------------------------------
      | CT1 = ControlType Tank 1
      | F1 = Fill Tank 1
      | E1 = Empty Tank 1
      | MR1 = Manual Reference Tank1
      | T1 = Temperature Tank 1
      | EB1 = Emergency Button Tank 1
      | LL1 = Liquid Level 1
  note: Inputs For Tank3
  note: Inputs For Tank1
  CT1 : Inport
  MR1 : Inport  Port=2
  T1 : Inport  Port=3
  EB1 : Inport  Port=4
  CT2 : Inport  Port=5
  MR2 : Inport  Port=6
  T2 : Inport  Port=7
  EB2 : Inport  Port=8
  CT3 : Inport  Port=9
  F3 : Inport  Port=10
  E3 : Inport  Port=11
  T3 : Inport  Port=12
  EB3 : Inport  Port=13
  Tank1 : Subsystem
  Tank2 : Subsystem
  Tank3 : Subsystem
  LL1 : Outport
  LL2 : Outport  Port=2
  LL3 : Outport  Port=3
  wires:
  EB1/1 -> Tank1/4(EB1)
  Tank2/1(LL2) -> LL2/1, Tank3/7(LL2), Tank1/5(LL2)
  Tank3/1(LL3) -> LL3/1, Tank2/6(LL3), Tank1/6(LL3)
  EB2/1 -> Tank2/4(EB2)
  CT2/1 -> Tank2/1(CT2)
  MR1/1 -> Tank1/2(MR1)
  T1/1 -> Tank1/3(T1)
  Tank1/1(LL1) -> LL1/1, Tank3/6(LL1), Tank2/5(LL1)
  E3/1 -> Tank3/3(E3)
  T2/1 -> Tank2/3(T2)
  CT3/1 -> Tank3/1(CT3)
  F3/1 -> Tank3/2(F3)
  EB3/1 -> Tank3/5(EB3)
  T3/1 -> Tank3/4(T3)
  CT1/1 -> Tank1/1(CT1)
  MR2/1 -> Tank2/2(MR2)

== system c00011M_harness/M200 ==
  note: VALUES
      | ---------------------------------
      | ControlType = 1 | 2 | 3
      | FillTank = 0 | 1
      | EmptyTank = 0 | 1
      | ManualReference between 0 and 1
      | Tempreature between 0 and 100
      | EmergencyButton = 0 | 1
      | LiquidLevel between 0 and 1 (hmax)
  note: Inputs For Tank2
  note: NAMES
      | --------------------------------------------
      | CT1 = ControlType Tank 1
      | F1 = Fill Tank 1
      | E1 = Empty Tank 1
      | MR1 = Manual Reference Tank1
      | T1 = Temperature Tank 1
      | EB1 = Emergency Button Tank 1
      | LL1 = Liquid Level 1
  note: Inputs For Tank3
  note: Inputs For Tank1
  CT1 : Inport
  MR1 : Inport  Port=2
  T1 : Inport  Port=3
  EB1 : Inport  Port=4
  CT2 : Inport  Port=5
  MR2 : Inport  Port=6
  T2 : Inport  Port=7
  EB2 : Inport  Port=8
  CT3 : Inport  Port=9
  F3 : Inport  Port=10
  E3 : Inport  Port=11
  T3 : Inport  Port=12
  EB3 : Inport  Port=13
  Tank1 : Subsystem
  Tank2 : Subsystem
  Tank3 : Subsystem
  LL1 : Outport
  LL2 : Outport  Port=2
  LL3 : Outport  Port=3
  wires:
  EB1/1 -> Tank1/4(EB1)
  Tank2/1(LL2) -> LL2/1, Tank3/7(LL2), Tank1/5(LL2)
  Tank3/1(LL3) -> LL3/1, Tank2/6(LL3), Tank1/6(LL3)
  EB2/1 -> Tank2/4(EB2)
  CT2/1 -> Tank2/1(CT2)
  MR1/1 -> Tank1/2(MR1)
  T1/1 -> Tank1/3(T1)
  Tank1/1(LL1) -> LL1/1, Tank3/6(LL1), Tank2/5(LL1)
  E3/1 -> Tank3/3(E3)
  T2/1 -> Tank2/3(T2)
  CT3/1 -> Tank3/1(CT3)
  F3/1 -> Tank3/2(F3)
  EB3/1 -> Tank3/5(EB3)
  T3/1 -> Tank3/4(T3)
  CT1/1 -> Tank1/1(CT1)
  MR2/1 -> Tank2/2(MR2)

== system c00011M_harness/M201 ==
  note: VALUES
      | ---------------------------------
      | ControlType = 1 | 2 | 3
      | FillTank = 0 | 1
      | EmptyTank = 0 | 1
      | ManualReference between 0 and 1
      | Tempreature between 0 and 100
      | EmergencyButton = 0 | 1
      | LiquidLevel between 0 and 1 (hmax)
  note: Inputs For Tank2
  note: NAMES
      | --------------------------------------------
      | CT1 = ControlType Tank 1
      | F1 = Fill Tank 1
      | E1 = Empty Tank 1
      | MR1 = Manual Reference Tank1
      | T1 = Temperature Tank 1
      | EB1 = Emergency Button Tank 1
      | LL1 = Liquid Level 1
  note: Inputs For Tank3
  note: Inputs For Tank1
  CT1 : Inport
  MR1 : Inport  Port=2
  T1 : Inport  Port=3
  EB1 : Inport  Port=4
  CT2 : Inport  Port=5
  MR2 : Inport  Port=6
  T2 : Inport  Port=7
  EB2 : Inport  Port=8
  CT3 : Inport  Port=9
  F3 : Inport  Port=10
  E3 : Inport  Port=11
  T3 : Inport  Port=12
  EB3 : Inport  Port=13
  Tank1 : Subsystem
  Tank2 : Subsystem
  Tank3 : Subsystem
  LL1 : Outport
  LL2 : Outport  Port=2
  LL3 : Outport  Port=3
  wires:
  EB1/1 -> Tank1/4(EB1)
  Tank2/1(LL2) -> LL2/1, Tank3/7(LL2), Tank1/5(LL2)
  Tank3/1(LL3) -> LL3/1, Tank2/6(LL3), Tank1/6(LL3)
  EB2/1 -> Tank2/4(EB2)
  CT2/1 -> Tank2/1(CT2)
  MR1/1 -> Tank1/2(MR1)
  T1/1 -> Tank1/3(T1)
  Tank1/1(LL1) -> LL1/1, Tank3/6(LL1), Tank2/5(LL1)
  E3/1 -> Tank3/3(E3)
  T2/1 -> Tank2/3(T2)
  CT3/1 -> Tank3/1(CT3)
  F3/1 -> Tank3/2(F3)
  EB3/1 -> Tank3/5(EB3)
  T3/1 -> Tank3/4(T3)
  CT1/1 -> Tank1/1(CT1)
  MR2/1 -> Tank2/2(MR2)

== system c00011M_harness/M202 ==
  note: VALUES
      | ---------------------------------
      | ControlType = 1 | 2 | 3
      | FillTank = 0 | 1
      | EmptyTank = 0 | 1
      | ManualReference between 0 and 1
      | Tempreature between 0 and 100
      | EmergencyButton = 0 | 1
      | LiquidLevel between 0 and 1 (hmax)
  note: Inputs For Tank2
  note: NAMES
      | --------------------------------------------
      | CT1 = ControlType Tank 1
      | F1 = Fill Tank 1
      | E1 = Empty Tank 1
      | MR1 = Manual Reference Tank1
      | T1 = Temperature Tank 1
      | EB1 = Emergency Button Tank 1
      | LL1 = Liquid Level 1
  note: Inputs For Tank3
  note: Inputs For Tank1
  CT1 : Inport
  MR1 : Inport  Port=2
  T1 : Inport  Port=3
  EB1 : Inport  Port=4
  CT2 : Inport  Port=5
  MR2 : Inport  Port=6
  T2 : Inport  Port=7
  EB2 : Inport  Port=8
  CT3 : Inport  Port=9
  F3 : Inport  Port=10
  E3 : Inport  Port=11
  T3 : Inport  Port=12
  EB3 : Inport  Port=13
  Tank1 : Subsystem
  Tank2 : Subsystem
  Tank3 : Subsystem
  LL1 : Outport
  LL2 : Outport  Port=2
  LL3 : Outport  Port=3
  wires:
  EB1/1 -> Tank1/4(EB1)
  Tank2/1(LL2) -> LL2/1, Tank3/7(LL2), Tank1/5(LL2)
  Tank3/1(LL3) -> LL3/1, Tank2/6(LL3), Tank1/6(LL3)
  EB2/1 -> Tank2/4(EB2)
  CT2/1 -> Tank2/1(CT2)
  MR1/1 -> Tank1/2(MR1)
  T1/1 -> Tank1/3(T1)
  Tank1/1(LL1) -> LL1/1, Tank3/6(LL1), Tank2/5(LL1)
  E3/1 -> Tank3/3(E3)
  T2/1 -> Tank2/3(T2)
  CT3/1 -> Tank3/1(CT3)
  F3/1 -> Tank3/2(F3)
  EB3/1 -> Tank3/5(EB3)
  T3/1 -> Tank3/4(T3)
  CT1/1 -> Tank1/1(CT1)
  MR2/1 -> Tank2/2(MR2)

== system c00011M_harness/M203 ==
  note: VALUES
      | ---------------------------------
      | ControlType = 1 | 2 | 3
      | FillTank = 0 | 1
      | EmptyTank = 0 | 1
      | ManualReference between 0 and 1
      | Tempreature between 0 and 100
      | EmergencyButton = 0 | 1
      | LiquidLevel between 0 and 1 (hmax)
  note: Inputs For Tank2
  note: NAMES
      | --------------------------------------------
      | CT1 = ControlType Tank 1
      | F1 = Fill Tank 1
      | E1 = Empty Tank 1
      | MR1 = Manual Reference Tank1
      | T1 = Temperature Tank 1
      | EB1 = Emergency Button Tank 1
      | LL1 = Liquid Level 1
  note: Inputs For Tank3
  note: Inputs For Tank1
  CT1 : Inport
  MR1 : Inport  Port=2
  T1 : Inport  Port=3
  EB1 : Inport  Port=4
  CT2 : Inport  Port=5
  MR2 : Inport  Port=6
  T2 : Inport  Port=7
  EB2 : Inport  Port=8
  CT3 : Inport  Port=9
  F3 : Inport  Port=10
  E3 : Inport  Port=11
  T3 : Inport  Port=12
  EB3 : Inport  Port=13
  Tank1 : Subsystem
  Tank2 : Subsystem
  Tank3 : Subsystem
  LL1 : Outport
  LL2 : Outport  Port=2
  LL3 : Outport  Port=3
  wires:
  EB1/1 -> Tank1/4(EB1)
  Tank2/1(LL2) -> LL2/1, Tank3/7(LL2), Tank1/5(LL2)
  Tank3/1(LL3) -> LL3/1, Tank2/6(LL3), Tank1/6(LL3)
  EB2/1 -> Tank2/4(EB2)
  CT2/1 -> Tank2/1(CT2)
  MR1/1 -> Tank1/2(MR1)
  T1/1 -> Tank1/3(T1)
  Tank1/1(LL1) -> LL1/1, Tank3/6(LL1), Tank2/5(LL1)
  E3/1 -> Tank3/3(E3)
  T2/1 -> Tank2/3(T2)
  CT3/1 -> Tank3/1(CT3)
  F3/1 -> Tank3/2(F3)
  EB3/1 -> Tank3/5(EB3)
  T3/1 -> Tank3/4(T3)
  CT1/1 -> Tank1/1(CT1)
  MR2/1 -> Tank2/2(MR2)

== system c00011M_harness/M204 ==
  note: VALUES
      | ---------------------------------
      | ControlType = 1 | 2 | 3
      | FillTank = 0 | 1
      | EmptyTank = 0 | 1
      | ManualReference between 0 and 1
      | Tempreature between 0 and 100
      | EmergencyButton = 0 | 1
      | LiquidLevel between 0 and 1 (hmax)
  note: Inputs For Tank2
  note: NAMES
      | --------------------------------------------
      | CT1 = ControlType Tank 1
      | F1 = Fill Tank 1
      | E1 = Empty Tank 1
      | MR1 = Manual Reference Tank1
      | T1 = Temperature Tank 1
      | EB1 = Emergency Button Tank 1
      | LL1 = Liquid Level 1
  note: Inputs For Tank3
  note: Inputs For Tank1
  CT1 : Inport
  MR1 : Inport  Port=2
  T1 : Inport  Port=3
  EB1 : Inport  Port=4
  CT2 : Inport  Port=5
  MR2 : Inport  Port=6
  T2 : Inport  Port=7
  EB2 : Inport  Port=8
  CT3 : Inport  Port=9
  F3 : Inport  Port=10
  E3 : Inport  Port=11
  T3 : Inport  Port=12
  EB3 : Inport  Port=13
  Tank1 : Subsystem
  Tank2 : Subsystem
  Tank3 : Subsystem
  LL1 : Outport
  LL2 : Outport  Port=2
  LL3 : Outport  Port=3
  wires:
  EB1/1 -> Tank1/4(EB1)
  Tank2/1(LL2) -> LL2/1, Tank3/7(LL2), Tank1/5(LL2)
  Tank3/1(LL3) -> LL3/1, Tank2/6(LL3), Tank1/6(LL3)
  EB2/1 -> Tank2/4(EB2)
  CT2/1 -> Tank2/1(CT2)
  MR1/1 -> Tank1/2(MR1)
  T1/1 -> Tank1/3(T1)
  Tank1/1(LL1) -> LL1/1, Tank3/6(LL1), Tank2/5(LL1)
  E3/1 -> Tank3/3(E3)
  T2/1 -> Tank2/3(T2)
  CT3/1 -> Tank3/1(CT3)
  F3/1 -> Tank3/2(F3)
  EB3/1 -> Tank3/5(EB3)
  T3/1 -> Tank3/4(T3)
  CT1/1 -> Tank1/1(CT1)
  MR2/1 -> Tank2/2(MR2)

== system c00011M_harness/M205 ==
  note: VALUES
      | ---------------------------------
      | ControlType = 1 | 2 | 3
      | FillTank = 0 | 1
      | EmptyTank = 0 | 1
      | ManualReference between 0 and 1
      | Tempreature between 0 and 100
      | EmergencyButton = 0 | 1
      | LiquidLevel between 0 and 1 (hmax)
  note: Inputs For Tank2
  note: NAMES
      | --------------------------------------------
      | CT1 = ControlType Tank 1
      | F1 = Fill Tank 1
      | E1 = Empty Tank 1
      | MR1 = Manual Reference Tank1
      | T1 = Temperature Tank 1
      | EB1 = Emergency Button Tank 1
      | LL1 = Liquid Level 1
  note: Inputs For Tank3
  note: Inputs For Tank1
  CT1 : Inport
  MR1 : Inport  Port=2
  T1 : Inport  Port=3
  EB1 : Inport  Port=4
  CT2 : Inport  Port=5
  MR2 : Inport  Port=6
  T2 : Inport  Port=7
  EB2 : Inport  Port=8
  CT3 : Inport  Port=9
  F3 : Inport  Port=10
  E3 : Inport  Port=11
  T3 : Inport  Port=12
  EB3 : Inport  Port=13
  Tank1 : Subsystem
  Tank2 : Subsystem
  Tank3 : Subsystem
  LL1 : Outport
  LL2 : Outport  Port=2
  LL3 : Outport  Port=3
  wires:
  EB1/1 -> Tank1/4(EB1)
  Tank2/1(LL2) -> LL2/1, Tank3/7(LL2), Tank1/5(LL2)
  Tank3/1(LL3) -> LL3/1, Tank2/6(LL3), Tank1/6(LL3)
  EB2/1 -> Tank2/4(EB2)
  CT2/1 -> Tank2/1(CT2)
  MR1/1 -> Tank1/2(MR1)
  T1/1 -> Tank1/3(T1)
  Tank1/1(LL1) -> LL1/1, Tank3/6(LL1), Tank2/5(LL1)
  E3/1 -> Tank3/3(E3)
  T2/1 -> Tank2/3(T2)
  CT3/1 -> Tank3/1(CT3)
  F3/1 -> Tank3/2(F3)
  EB3/1 -> Tank3/5(EB3)
  T3/1 -> Tank3/4(T3)
  CT1/1 -> Tank1/1(CT1)
  MR2/1 -> Tank2/2(MR2)

== system c00011M_harness/M206 ==
  note: VALUES
      | ---------------------------------
      | ControlType = 1 | 2 | 3
      | FillTank = 0 | 1
      | EmptyTank = 0 | 1
      | ManualReference between 0 and 1
      | Tempreature between 0 and 100
      | EmergencyButton = 0 | 1
      | LiquidLevel between 0 and 1 (hmax)
  note: Inputs For Tank2
  note: NAMES
      | --------------------------------------------
      | CT1 = ControlType Tank 1
      | F1 = Fill Tank 1
      | E1 = Empty Tank 1
      | MR1 = Manual Reference Tank1
      | T1 = Temperature Tank 1
      | EB1 = Emergency Button Tank 1
      | LL1 = Liquid Level 1
  note: Inputs For Tank3
  note: Inputs For Tank1
  CT1 : Inport
  MR1 : Inport  Port=2
  T1 : Inport  Port=3
  EB1 : Inport  Port=4
  CT2 : Inport  Port=5
  MR2 : Inport  Port=6
  T2 : Inport  Port=7
  EB2 : Inport  Port=8
  CT3 : Inport  Port=9
  F3 : Inport  Port=10
  E3 : Inport  Port=11
  T3 : Inport  Port=12
  EB3 : Inport  Port=13
  Tank1 : Subsystem
  Tank2 : Subsystem
  Tank3 : Subsystem
  LL1 : Outport
  LL2 : Outport  Port=2
  LL3 : Outport  Port=3
  wires:
  EB1/1 -> Tank1/4(EB1)
  Tank2/1(LL2) -> LL2/1, Tank3/7(LL2), Tank1/5(LL2)
  Tank3/1(LL3) -> LL3/1, Tank2/6(LL3), Tank1/6(LL3)
  EB2/1 -> Tank2/4(EB2)
  CT2/1 -> Tank2/1(CT2)
  MR1/1 -> Tank1/2(MR1)
  T1/1 -> Tank1/3(T1)
  Tank1/1(LL1) -> LL1/1, Tank3/6(LL1), Tank2/5(LL1)
  E3/1 -> Tank3/3(E3)
  T2/1 -> Tank2/3(T2)
  CT3/1 -> Tank3/1(CT3)
  F3/1 -> Tank3/2(F3)
  EB3/1 -> Tank3/5(EB3)
  T3/1 -> Tank3/4(T3)
  CT1/1 -> Tank1/1(CT1)
  MR2/1 -> Tank2/2(MR2)

== system c00011M_harness/M207 ==
  note: VALUES
      | ---------------------------------
      | ControlType = 1 | 2 | 3
      | FillTank = 0 | 1
      | EmptyTank = 0 | 1
      | ManualReference between 0 and 1
      | Tempreature between 0 and 100
      | EmergencyButton = 0 | 1
      | LiquidLevel between 0 and 1 (hmax)
  note: Inputs For Tank2
  note: NAMES
      | --------------------------------------------
      | CT1 = ControlType Tank 1
      | F1 = Fill Tank 1
      | E1 = Empty Tank 1
      | MR1 = Manual Reference Tank1
      | T1 = Temperature Tank 1
      | EB1 = Emergency Button Tank 1
      | LL1 = Liquid Level 1
  note: Inputs For Tank3
  note: Inputs For Tank1
  CT1 : Inport
  MR1 : Inport  Port=2
  T1 : Inport  Port=3
  EB1 : Inport  Port=4
  CT2 : Inport  Port=5
  MR2 : Inport  Port=6
  T2 : Inport  Port=7
  EB2 : Inport  Port=8
  CT3 : Inport  Port=9
  F3 : Inport  Port=10
  E3 : Inport  Port=11
  T3 : Inport  Port=12
  EB3 : Inport  Port=13
  Tank1 : Subsystem
  Tank2 : Subsystem
  Tank3 : Subsystem
  LL1 : Outport
  LL2 : Outport  Port=2
  LL3 : Outport  Port=3
  wires:
  EB1/1 -> Tank1/4(EB1)
  Tank2/1(LL2) -> LL2/1, Tank3/7(LL2), Tank1/5(LL2)
  Tank3/1(LL3) -> LL3/1, Tank2/6(LL3), Tank1/6(LL3)
  EB2/1 -> Tank2/4(EB2)
  CT2/1 -> Tank2/1(CT2)
  MR1/1 -> Tank1/2(MR1)
  T1/1 -> Tank1/3(T1)
  Tank1/1(LL1) -> LL1/1, Tank3/6(LL1), Tank2/5(LL1)
  E3/1 -> Tank3/3(E3)
  T2/1 -> Tank2/3(T2)
  CT3/1 -> Tank3/1(CT3)
  F3/1 -> Tank3/2(F3)
  EB3/1 -> Tank3/5(EB3)
  T3/1 -> Tank3/4(T3)
  CT1/1 -> Tank1/1(CT1)
  MR2/1 -> Tank2/2(MR2)

== system c00011M_harness/M208 ==
  note: VALUES
      | ---------------------------------
      | ControlType = 1 | 2 | 3
      | FillTank = 0 | 1
      | EmptyTank = 0 | 1
      | ManualReference between 0 and 1
      | Tempreature between 0 and 100
      | EmergencyButton = 0 | 1
      | LiquidLevel between 0 and 1 (hmax)
  note: Inputs For Tank2
  note: NAMES
      | --------------------------------------------
      | CT1 = ControlType Tank 1
      | F1 = Fill Tank 1
      | E1 = Empty Tank 1
      | MR1 = Manual Reference Tank1
      | T1 = Temperature Tank 1
      | EB1 = Emergency Button Tank 1
      | LL1 = Liquid Level 1
  note: Inputs For Tank3
  note: Inputs For Tank1
  CT1 : Inport
  MR1 : Inport  Port=2
  T1 : Inport  Port=3
  EB1 : Inport  Port=4
  CT2 : Inport  Port=5
  MR2 : Inport  Port=6
  T2 : Inport  Port=7
  EB2 : Inport  Port=8
  CT3 : Inport  Port=9
  F3 : Inport  Port=10
  E3 : Inport  Port=11
  T3 : Inport  Port=12
  EB3 : Inport  Port=13
  Tank1 : Subsystem
  Tank2 : Subsystem
  Tank3 : Subsystem
  LL1 : Outport
  LL2 : Outport  Port=2
  LL3 : Outport  Port=3
  wires:
  EB1/1 -> Tank1/4(EB1)
  Tank2/1(LL2) -> LL2/1, Tank3/7(LL2), Tank1/5(LL2)
  Tank3/1(LL3) -> LL3/1, Tank2/6(LL3), Tank1/6(LL3)
  EB2/1 -> Tank2/4(EB2)
  CT2/1 -> Tank2/1(CT2)
  MR1/1 -> Tank1/2(MR1)
  T1/1 -> Tank1/3(T1)
  Tank1/1(LL1) -> LL1/1, Tank3/6(LL1), Tank2/5(LL1)
  E3/1 -> Tank3/3(E3)
  T2/1 -> Tank2/3(T2)
  CT3/1 -> Tank3/1(CT3)
  F3/1 -> Tank3/2(F3)
  EB3/1 -> Tank3/5(EB3)
  T3/1 -> Tank3/4(T3)
  CT1/1 -> Tank1/1(CT1)
  MR2/1 -> Tank2/2(MR2)

== system c00011M_harness/M209 ==
  note: VALUES
      | ---------------------------------
      | ControlType = 1 | 2 | 3
      | FillTank = 0 | 1
      | EmptyTank = 0 | 1
      | ManualReference between 0 and 1
      | Tempreature between 0 and 100
      | EmergencyButton = 0 | 1
      | LiquidLevel between 0 and 1 (hmax)
  note: Inputs For Tank2
  note: NAMES
      | --------------------------------------------
      | CT1 = ControlType Tank 1
      | F1 = Fill Tank 1
      | E1 = Empty Tank 1
      | MR1 = Manual Reference Tank1
      | T1 = Temperature Tank 1
      | EB1 = Emergency Button Tank 1
      | LL1 = Liquid Level 1
  note: Inputs For Tank3
  note: Inputs For Tank1
  CT1 : Inport
  MR1 : Inport  Port=2
  T1 : Inport  Port=3
  EB1 : Inport  Port=4
  CT2 : Inport  Port=5
  MR2 : Inport  Port=6
  T2 : Inport  Port=7
  EB2 : Inport  Port=8
  CT3 : Inport  Port=9
  F3 : Inport  Port=10
  E3 : Inport  Port=11
  T3 : Inport  Port=12
  EB3 : Inport  Port=13
  Tank1 : Subsystem
  Tank2 : Subsystem
  Tank3 : Subsystem
  LL1 : Outport
  LL2 : Outport  Port=2
  LL3 : Outport  Port=3
  wires:
  EB1/1 -> Tank1/4(EB1)
  Tank2/1(LL2) -> LL2/1, Tank3/7(LL2), Tank1/5(LL2)
  Tank3/1(LL3) -> LL3/1, Tank2/6(LL3), Tank1/6(LL3)
  EB2/1 -> Tank2/4(EB2)
  CT2/1 -> Tank2/1(CT2)
  MR1/1 -> Tank1/2(MR1)
  T1/1 -> Tank1/3(T1)
  Tank1/1(LL1) -> LL1/1, Tank3/6(LL1), Tank2/5(LL1)
  E3/1 -> Tank3/3(E3)
  T2/1 -> Tank2/3(T2)
  CT3/1 -> Tank3/1(CT3)
  F3/1 -> Tank3/2(F3)
  EB3/1 -> Tank3/5(EB3)
  T3/1 -> Tank3/4(T3)
  CT1/1 -> Tank1/1(CT1)
  MR2/1 -> Tank2/2(MR2)

== system c00011M_harness/M222 ==
  note: VALUES
      | ---------------------------------
      | ControlType = 1 | 2 | 3
      | FillTank = 0 | 1
      | EmptyTank = 0 | 1
      | ManualReference between 0 and 1
      | Tempreature between 0 and 100
      | EmergencyButton = 0 | 1
      | LiquidLevel between 0 and 1 (hmax)
  note: Inputs For Tank2
  note: NAMES
      | --------------------------------------------
      | CT1 = ControlType Tank 1
      | F1 = Fill Tank 1
      | E1 = Empty Tank 1
      | MR1 = Manual Reference Tank1
      | T1 = Temperature Tank 1
      | EB1 = Emergency Button Tank 1
      | LL1 = Liquid Level 1
  note: Inputs For Tank3
  note: Inputs For Tank1
  CT1 : Inport
  MR1 : Inport  Port=2
  T1 : Inport  Port=3
  EB1 : Inport  Port=4
  CT2 : Inport  Port=5
  MR2 : Inport  Port=6
  T2 : Inport  Port=7
  EB2 : Inport  Port=8
  CT3 : Inport  Port=9
  F3 : Inport  Port=10
  E3 : Inport  Port=11
  T3 : Inport  Port=12
  EB3 : Inport  Port=13
  Tank1 : Subsystem
  Tank2 : Subsystem
  Tank3 : Subsystem
  LL1 : Outport
  LL2 : Outport  Port=2
  LL3 : Outport  Port=3
  wires:
  EB1/1 -> Tank1/4(EB1)
  Tank2/1(LL2) -> LL2/1, Tank3/7(LL2), Tank1/5(LL2)
  Tank3/1(LL3) -> LL3/1, Tank2/6(LL3), Tank1/6(LL3)
  EB2/1 -> Tank2/4(EB2)
  CT2/1 -> Tank2/1(CT2)
  MR1/1 -> Tank1/2(MR1)
  T1/1 -> Tank1/3(T1)
  Tank1/1(LL1) -> LL1/1, Tank3/6(LL1), Tank2/5(LL1)
  E3/1 -> Tank3/3(E3)
  T2/1 -> Tank2/3(T2)
  CT3/1 -> Tank3/1(CT3)
  F3/1 -> Tank3/2(F3)
  EB3/1 -> Tank3/5(EB3)
  T3/1 -> Tank3/4(T3)
  CT1/1 -> Tank1/1(CT1)
  MR2/1 -> Tank2/2(MR2)

== system c00011M_harness/M223 ==
  note: VALUES
      | ---------------------------------
      | ControlType = 1 | 2 | 3
      | FillTank = 0 | 1
      | EmptyTank = 0 | 1
      | ManualReference between 0 and 1
      | Tempreature between 0 and 100
      | EmergencyButton = 0 | 1
      | LiquidLevel between 0 and 1 (hmax)
  note: Inputs For Tank2
  note: NAMES
      | --------------------------------------------
      | CT1 = ControlType Tank 1
      | F1 = Fill Tank 1
      | E1 = Empty Tank 1
      | MR1 = Manual Reference Tank1
      | T1 = Temperature Tank 1
      | EB1 = Emergency Button Tank 1
      | LL1 = Liquid Level 1
  note: Inputs For Tank3
  note: Inputs For Tank1
  CT1 : Inport
  MR1 : Inport  Port=2
  T1 : Inport  Port=3
  EB1 : Inport  Port=4
  CT2 : Inport  Port=5
  MR2 : Inport  Port=6
  T2 : Inport  Port=7
  EB2 : Inport  Port=8
  CT3 : Inport  Port=9
  F3 : Inport  Port=10
  E3 : Inport  Port=11
  T3 : Inport  Port=12
  EB3 : Inport  Port=13
  Tank1 : Subsystem
  Tank2 : Subsystem
  Tank3 : Subsystem
  LL1 : Outport
  LL2 : Outport  Port=2
  LL3 : Outport  Port=3
  wires:
  EB1/1 -> Tank1/4(EB1)
  Tank2/1(LL2) -> LL2/1, Tank3/7(LL2), Tank1/5(LL2)
  Tank3/1(LL3) -> LL3/1, Tank2/6(LL3), Tank1/6(LL3)
  EB2/1 -> Tank2/4(EB2)
  CT2/1 -> Tank2/1(CT2)
  MR1/1 -> Tank1/2(MR1)
  T1/1 -> Tank1/3(T1)
  Tank1/1(LL1) -> LL1/1, Tank3/6(LL1), Tank2/5(LL1)
  E3/1 -> Tank3/3(E3)
  T2/1 -> Tank2/3(T2)
  CT3/1 -> Tank3/1(CT3)
  F3/1 -> Tank3/2(F3)
  EB3/1 -> Tank3/5(EB3)
  T3/1 -> Tank3/4(T3)
  CT1/1 -> Tank1/1(CT1)
  MR2/1 -> Tank2/2(MR2)

== system c00011M_harness/M224 ==
  note: VALUES
      | ---------------------------------
      | ControlType = 1 | 2 | 3
      | FillTank = 0 | 1
      | EmptyTank = 0 | 1
      | ManualReference between 0 and 1
      | Tempreature between 0 and 100
      | EmergencyButton = 0 | 1
      | LiquidLevel between 0 and 1 (hmax)
  note: Inputs For Tank2
  note: NAMES
      | --------------------------------------------
      | CT1 = ControlType Tank 1
      | F1 = Fill Tank 1
      | E1 = Empty Tank 1
      | MR1 = Manual Reference Tank1
      | T1 = Temperature Tank 1
      | EB1 = Emergency Button Tank 1
      | LL1 = Liquid Level 1
  note: Inputs For Tank3
  note: Inputs For Tank1
  CT1 : Inport
  MR1 : Inport  Port=2
  T1 : Inport  Port=3
  EB1 : Inport  Port=4
  CT2 : Inport  Port=5
  MR2 : Inport  Port=6
  T2 : Inport  Port=7
  EB2 : Inport  Port=8
  CT3 : Inport  Port=9
  F3 : Inport  Port=10
  E3 : Inport  Port=11
  T3 : Inport  Port=12
  EB3 : Inport  Port=13
  Tank1 : Subsystem
  Tank2 : Subsystem
  Tank3 : Subsystem
  LL1 : Outport
  LL2 : Outport  Port=2
  LL3 : Outport  Port=3
  wires:
  EB1/1 -> Tank1/4(EB1)
  Tank2/1(LL2) -> LL2/1, Tank3/7(LL2), Tank1/5(LL2)
  Tank3/1(LL3) -> LL3/1, Tank2/6(LL3), Tank1/6(LL3)
  EB2/1 -> Tank2/4(EB2)
  CT2/1 -> Tank2/1(CT2)
  MR1/1 -> Tank1/2(MR1)
  T1/1 -> Tank1/3(T1)
  Tank1/1(LL1) -> LL1/1, Tank3/6(LL1), Tank2/5(LL1)
  E3/1 -> Tank3/3(E3)
  T2/1 -> Tank2/3(T2)
  CT3/1 -> Tank3/1(CT3)
  F3/1 -> Tank3/2(F3)
  EB3/1 -> Tank3/5(EB3)
  T3/1 -> Tank3/4(T3)
  CT1/1 -> Tank1/1(CT1)
  MR2/1 -> Tank2/2(MR2)
